simulink model "Modelo_V3_vertical"  (R2021b)
settings: Solver=FixedStepAuto  StartTime=0.0  StopTime=20  FixedStep=10^-3  RelTol=1e-3
values from neighbouring files (symbols this model uses):
  C = 4000    [varglobal.m]
  Kf = 20000    [varglobal.m]
  Kp = 200000    [varglobal.m]
  Kr = 20000    [varglobal.m]
undefined symbols (not defined in the file or in its folder): eqmovimento, lombadatravessia, Transformador, TransformadorT
libraries: simulink_extras x1
settings Model: Creator=Vilson Wenis Belle  LastModifiedBy=usuario
settings SolverCC: AlgebraicLoopSolver=TrustRegion

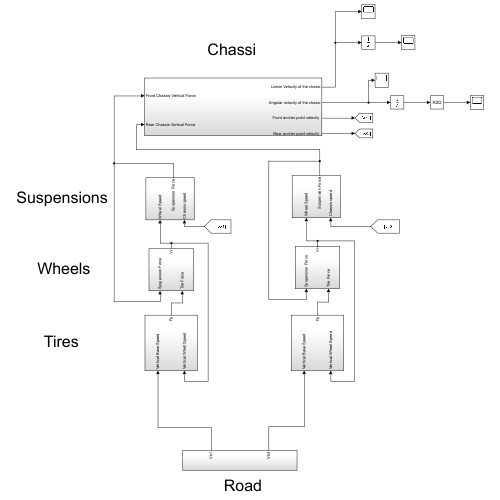
[thumbnail: Simulink's stored preview of the top-level diagram]
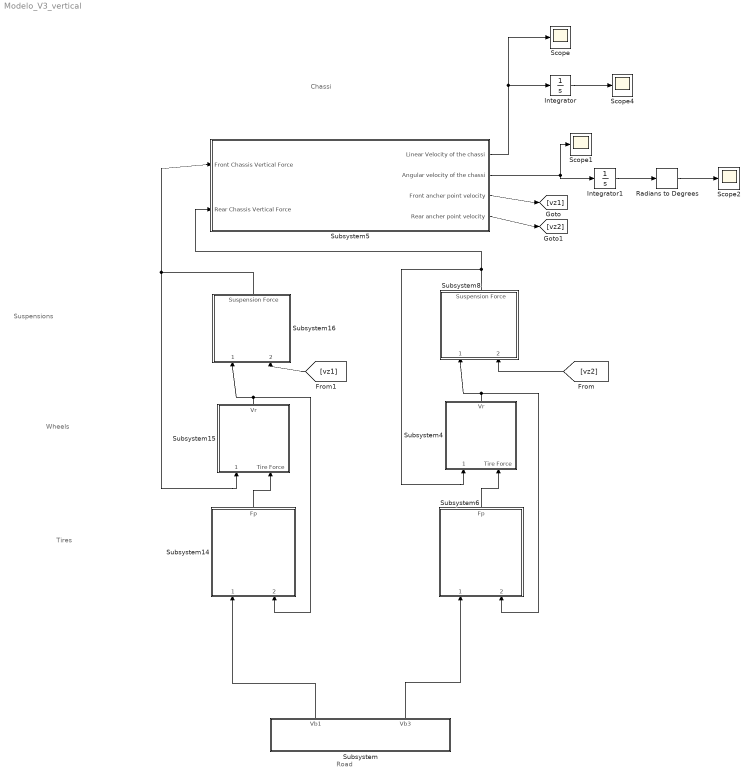
== system Modelo_V3_vertical ==
  note: Tires
  note: Road
  note: Suspensions
  note: Wheels
  note: Chassi
  Integrator : Integrator
  Integrator1 : Integrator
  Radians to Degrees : simulink_extras/Transformations/Radians to Degrees
  Scope{,1..2,4} (4 alike) : Scope
  Subsystem : Subsystem
  Subsystem14 : Subsystem
  Subsystem15 : Subsystem
  Subsystem16 : Subsystem
  Subsystem4 : Subsystem
  Subsystem5 : Subsystem
  Subsystem6 : Subsystem
  Subsystem8 : Subsystem
  wires:
  Subsystem4/1(Vr) -> Subsystem8/1(Wheel Speed), Subsystem6/2(Vertical Wheel Speed)
  Subsystem6/1(Fp) -> Subsystem4/2(Tire Force)
  Subsystem15/1(Vr) -> Subsystem16/1(Wheel Speed), Subsystem14/2(Vertical Whell Speed)
  Subsystem14/1(Fp) -> Subsystem15/2(Tire Force)
  Subsystem16/1(Suspension Force) -> Subsystem5/1(Front Chassis Vertical Force), Subsystem15/1(Suspension Force)
  Subsystem8/1(Suspension Force) -> Subsystem4/1(Suspension Force), Subsystem5/2(Rear Chassis Vertical Force)
  Subsystem5/1(Linear Velocity of the chassi) -> Scope/1, Integrator/1
  Integrator/1 -> Scope4/1
  Subsystem/2(Vb3) -> Subsystem6/1(Vertical Base Speed)
  Subsystem5/2(Angular velocity of the chassi) -> Scope1/1, Integrator1/1
  Subsystem/1(Vb1) -> Subsystem14/1(Vertical Base Speed)
  Subsystem5/3("Front ancher point velocity ") -> [vz1]
  Subsystem5/4("Rear ancher point velocity ") -> [vz2]
  [vz2] -> Subsystem8/2(Chassis speed)
  [vz1] -> Subsystem16/2(Chassis speed)
  Integrator1/1 -> Radians to Degrees/1
  Radians to Degrees/1 -> Scope2/1

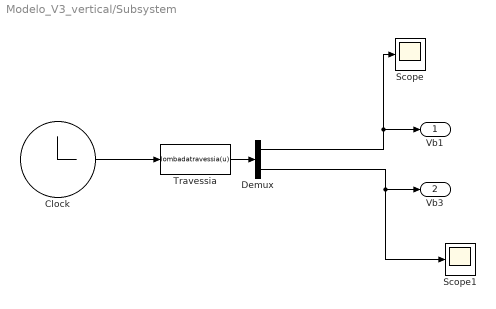
== system Modelo_V3_vertical/Subsystem ==
  Clock : Clock
      settings: Decimation=1000
  Demux : Demux  Outputs=2
  Scope : Scope
  Scope1 : Scope
  Travessia : MATLABFcn  MATLABFcn=lombadatravessia(u)  OutputDimensions=2
  Vb1 : Outport
  Vb3 : Outport  Port=2
  wires:
  Clock/1 -> Travessia/1
  Demux/1 -> Vb1/1, Scope/1
  Demux/2 -> Vb3/1, Scope1/1
  Travessia/1 -> Demux/1

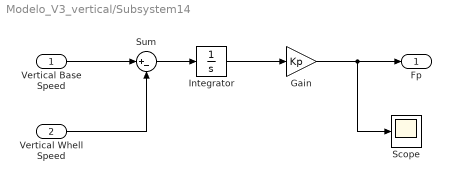
== system Modelo_V3_vertical/Subsystem14 ==
  Vertical Base Speed : Inport
  Vertical Whell Speed : Inport  Port=2
  Gain : Gain  Gain=Kp
  Integrator : Integrator
  Scope : Scope
  Sum : Sum  Inputs=|+-
  Fp : Outport
  wires:
  Vertical Whell Speed/1 -> Sum/2
  Vertical Base Speed/1 -> Sum/1
  Sum/1 -> Integrator/1
  Integrator/1 -> Gain/1
  Gain/1 -> Scope/1, Fp/1

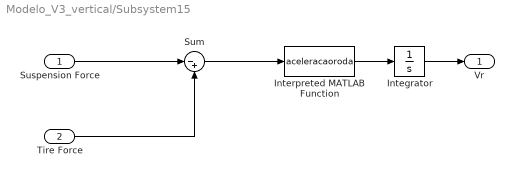
== system Modelo_V3_vertical/Subsystem15 ==
  Suspension Force : Inport
  Tire Force : Inport  Port=2
  Integrator : Integrator
  Interpreted MATLAB Function : MATLABFcn  MATLABFcn=aceleracaoroda  OutputDimensions=1
  Sum : Sum  Inputs=|-+
  Vr : Outport
  wires:
  Suspension Force/1 -> Sum/1
  Tire Force/1 -> Sum/2
  Integrator/1 -> Vr/1
  Sum/1 -> Interpreted MATLAB Function/1
  Interpreted MATLAB Function/1 -> Integrator/1

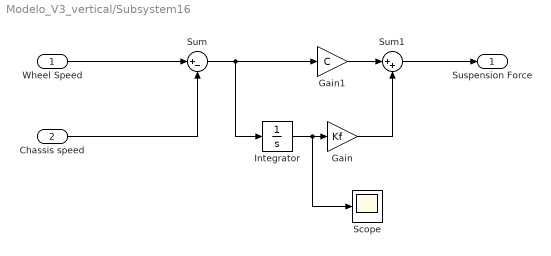
== system Modelo_V3_vertical/Subsystem16 ==
  Wheel Speed : Inport
  Chassis speed : Inport  Port=2
  Gain : Gain  Gain=Kf
  Gain1 : Gain  Gain=C
  Integrator : Integrator
  Scope : Scope
  Sum : Sum  Inputs=|+-
  Sum1 : Sum  Inputs=|++
  Suspension Force : Outport
  wires:
  Chassis speed/1 -> Sum/2
  Wheel Speed/1 -> Sum/1
  Sum/1 -> Gain1/1, Integrator/1
  Integrator/1 -> Scope/1, Gain/1
  Gain1/1 -> Sum1/1
  Gain/1 -> Sum1/2
  Sum1/1 -> Suspension Force/1

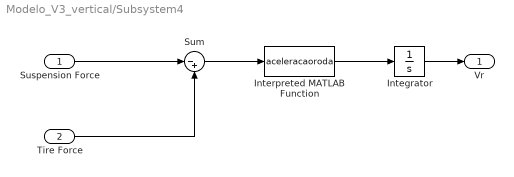
== system Modelo_V3_vertical/Subsystem4 ==
  Suspension Force : Inport
  Tire Force : Inport  Port=2
  Integrator : Integrator
  Interpreted MATLAB Function : MATLABFcn  MATLABFcn=aceleracaoroda  OutputDimensions=1
  Sum : Sum  Inputs=|-+
  Vr : Outport
  wires:
  Suspension Force/1 -> Sum/1
  Tire Force/1 -> Sum/2
  Integrator/1 -> Vr/1
  Sum/1 -> Interpreted MATLAB Function/1
  Interpreted MATLAB Function/1 -> Integrator/1

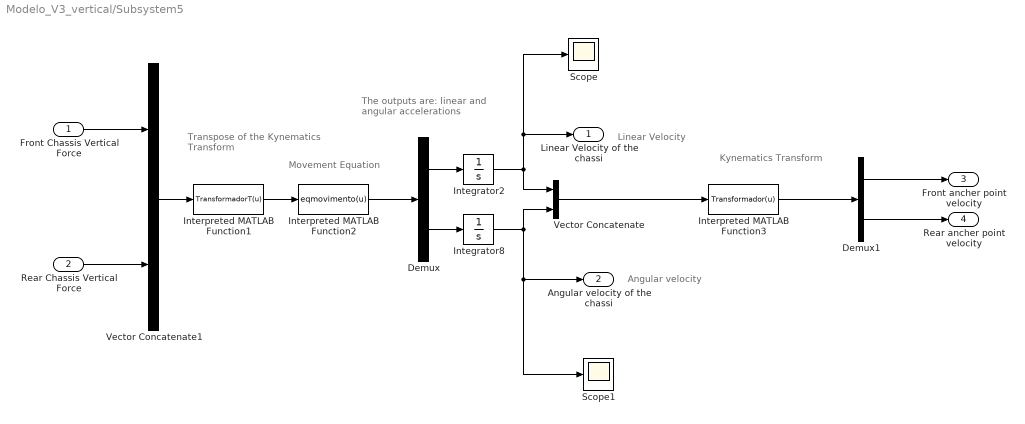
== system Modelo_V3_vertical/Subsystem5 ==
  note: Angular velocity
  note: Linear Velocity
  note: The outputs are: linear and
      | angular accelerations
  note: Transpose of the
      | Kynematics
      | Transform
  note: Movement Equation
  note: Kynematics
      | Transform
  Front Chassis Vertical Force : Inport
  Rear Chassis Vertical Force : Inport  Port=2
  Demux : Demux  Outputs=2
  Demux1 : Demux  Outputs=2
  Integrator2 : Integrator
  Integrator8 : Integrator
  Interpreted MATLAB Function1 : MATLABFcn  MATLABFcn=TransformadorT(u)  OutputDimensions=2
  Interpreted MATLAB Function2 : MATLABFcn  MATLABFcn=eqmovimento(u)  OutputDimensions=2
  Interpreted MATLAB Function3 : MATLABFcn  MATLABFcn=Transformador(u)  OutputDimensions=2
  Scope : Scope
  Scope1 : Scope
  Vector Concatenate : Concatenate
  Vector Concatenate1 : Concatenate
  Linear Velocity of the chassi : Outport
  Angular velocity of the chassi : Outport  Port=2
  "Front ancher point velocity " : Outport  Port=3
  "Rear ancher point velocity " : Outport  Port=4
  wires:
  Demux1/2 -> "Rear ancher point velocity "/1
  Demux1/1 -> "Front ancher point velocity "/1
  Vector Concatenate1/1 -> Interpreted MATLAB Function1/1
  Rear Chassis Vertical Force/1 -> Vector Concatenate1/2
  Front Chassis Vertical Force/1 -> Vector Concatenate1/1
  Interpreted MATLAB Function1/1 -> Interpreted MATLAB Function2/1
  Interpreted MATLAB Function2/1 -> Demux/1
  Demux/1 -> Integrator2/1
  Demux/2 -> Integrator8/1
  Integrator2/1 -> Vector Concatenate/1, Scope/1, Linear Velocity of the chassi/1
  Vector Concatenate/1 -> Interpreted MATLAB Function3/1
  Integrator8/1 -> Scope1/1, Angular velocity of the chassi/1, Vector Concatenate/2
  Interpreted MATLAB Function3/1 -> Demux1/1

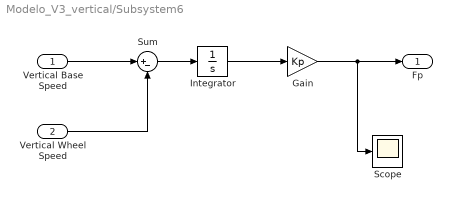
== system Modelo_V3_vertical/Subsystem6 ==
  Vertical Base Speed : Inport
  Vertical Wheel Speed : Inport  Port=2
  Gain : Gain  Gain=Kp
  Integrator : Integrator
  Scope : Scope
  Sum : Sum  Inputs=|+-
  Fp : Outport
  wires:
  Vertical Wheel Speed/1 -> Sum/2
  Vertical Base Speed/1 -> Sum/1
  Sum/1 -> Integrator/1
  Integrator/1 -> Gain/1
  Gain/1 -> Scope/1, Fp/1

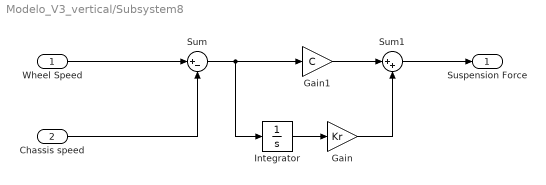
== system Modelo_V3_vertical/Subsystem8 ==
  Wheel Speed : Inport
  Chassis speed : Inport  Port=2
  Gain : Gain  Gain=Kr
  Gain1 : Gain  Gain=C
  Integrator : Integrator
  Sum : Sum  Inputs=|+-
  Sum1 : Sum  Inputs=|++
  Suspension Force : Outport
  wires:
  Chassis speed/1 -> Sum/2
  Wheel Speed/1 -> Sum/1
  Sum/1 -> Gain1/1, Integrator/1
  Integrator/1 -> Gain/1
  Gain1/1 -> Sum1/1
  Gain/1 -> Sum1/2
  Sum1/1 -> Suspension Force/1
